simulink subsystem "Controller"  (R2024b)
settings: Solver=VariableStepAuto  StartTime=0.0  StopTime=10.0  RelTol=1e-3
undefined symbols (not defined in the file or in its folder): flight_mode, Parameters, References
libraries: sharedtransform x13, eeGeneralControl x10, simulink x5, aerolibutil x2
(part 3 of 3)

== matlab function Controller/Subsystem/OLD/position_control + autonomous/If Action Subsystem/Attitude + Position FF control/MATLAB Function1 ==
  data: T_des output; p_ref input; att_dir_correction_from_pos_ output; v_ref input; a_ref input; K_pos input; K_pos_int input; K_vel input; K_acc input; pi input; vi input; ai input; q input; p_fb_int input; p_fb_out output
function [T_des, att_dir_correction_from_pos_, p_fb_out] = pos_FF_control(...
    p_ref, v_ref, a_ref, ...
    K_pos, K_pos_int, K_vel, K_acc,...
    pi, vi, ai, q,...
    p_fb_int)

%% inputs %%
p_ref_ = p_ref(1:3,1);      %[m] reference position (in inertial frame)
v_ref_ = v_ref(1:3,1);      %[m/s] reference velocity (in inertial frame)
a_ref_ = a_ref(1:3,1);      %[m/s2] reference acceleration (in inertial frame)
% psi_ref_ = psi_ref(1,1);    %[rad] reference heading

% J_ = J(1:3,1:3);            % moment of inertia matrix
% D_ = diag(D(1,1:3));        % drag coefficient
% g_ = g(1,1);                %[m/s2] acceleration due to gravity
K_pos_ = ...
    K_pos(1:3,1:3);     % position controller gains
K_pos_int_ = ...
    K_pos_int(1:3,1:3); % position controller integral gains
K_vel_ = ...
    K_vel(1:3,1:3);     % velocity controller gains
K_acc_ = ...
    K_acc(1:3,1:3);     % acceleration controller gains
% K_att_ = ...
%     K_att(1:3,1:3);     % attitude controller gains
% K_omega_ = ...
    % K_omega(1:3,1:3);   % body rate controller gains
% A_ = A(1:3,1:3);            % velocity-dependant drag coefficients
% B_ = B(1:3,1:3);            % omega-dependant drag coefficients
% k_h_ = k_h(1,1);            % constant for a quadratic velocity-dependent input disturbance

% q_ref_ = q_ref(1,1:4);      % reference attitude quaternian
% omega_ref_ = ...
%     omega_ref(1:3,1);       %[rad/s] reference body rates
% omega_dot_ref_ = ...
%     omega_dot_ref(1:3,1);   %[rad/s2] reference body rotational acceleration
% Tau_ref_ = Tau_ref(1:3,1);  %[N-m] reference torque
% T_ref_ = T_ref(1,1);        %[N] reference collective thrust

pi_ = pi(1:3,1);            %[m] estimated position (in inertial frame)
vi_ = vi(1:3,1);            %[m/s] estimated velocity (in inertial frame)
ai_ = ai(1:3,1);            %[m/s2] estimated acceleration (in inertial frame)
q_ = q(1,1:4);              %[qw qx qy qz] estimated quaternian attitude
% omega_ = omega(1:3,1);      %[rad/s] estimated body rotation rates
% tau_gyro_ = ...
    % tau_gyro(1:3,1);        %[N-m] estimated gyroscopic torque due to motor spin

p_fb_int_ = p_fb_int(1:3,1); %integral of the position feedback term  

%% outputs %%
% T_des = 0;                  %[N] desired thrust
% Tau_des = zeros(3,1);       %[N-m] desired torque
% p_fb = zeros(3,1);
% v_fb = zeros(3,1);
% a_fb_ = zeros(3,1);

% att_fb = zeros(3,1);
% omega_fb = zeros(3,1);
% omega_dot_des = zeros(3,1);
T_des = 0;
p_fb_out = zeros(3,1); %we will integrate this

%% Positon Control %%
MAX_XYZ_POS_ERR = 10.0;
MAX_XYZ_VEL_ERR = 5.0;
MAX_XYZ_ACC_ERR = 3;


%feedback control:
p_fb_ = (p_ref_ - pi_);
p_fb_out(:) = p_fb_(:);
p_fb_ = K_pos_ * (saturate_err_vec_(p_fb_, -MAX_XYZ_POS_ERR, MAX_XYZ_POS_ERR)) + K_pos_int_*p_fb_int_;

v_fb_ = (v_ref_ - vi_);
v_fb_ = K_vel_ * (saturate_err_vec_(v_fb_, -MAX_XYZ_VEL_ERR, MAX_XYZ_VEL_ERR));

a_fb_ = (a_ref_ - ai_);
a_fb_ = K_acc_ * (saturate_err_vec_(a_fb_, -MAX_XYZ_ACC_ERR, MAX_XYZ_ACC_ERR));

%feedback component:
att_dir_correction_from_pos_ = a_fb_ + v_fb_ + p_fb_; %from position controller

%thrust feedback:
T_des(1) = [att_dir_correction_from_pos_(1),att_dir_correction_from_pos_(2),att_dir_correction_from_pos_(3)]*lib.math.quatrotate(q_, [0;0;-1]);

end

function out = saturate_err_vec_(in, out_min, out_max)
    n = length(in);
    if ~isequal(length(out_min),n)
        out_min_ = out_min(1)*ones(1,n);
    else
        out_min_ = out_min(:)';
    end
    if ~isequal(length(out_max),n)
        out_max_ = out_max(1)*ones(1,n);
    else
        out_max_ = out_max(:)';
    end
    out = zeros(n,1);
    for i = 1:n
        out(i) = saturate_err__(in(i), out_min_(i), out_max_(i));
    end

    function out = saturate_err__(in, out_min, out_max)
        in_ = in(1);
        if in_ > out_max
            out = 1;
            return;
        elseif in_ < out_min
            out = -1;
            return;
        else
            out = in_ / (out_max - out_min);
            return;
        end
    end
end
function out = sqrt_ctr_(in)
    out = sign(in) .*sqrt(abs(in));
end
function out = nthrt_ctr_(in)
    out = sign(in) .*nthroot(abs(in),3);
end

== matlab function Controller/Subsystem/OLD/position_control + autonomous/If Action Subsystem/Attitude + Position FF control/MATLAB Function2 ==
  data: omega_dot_des output; att_dir_correction_from_pos input; q_ref input; omega_ref input; K_att input; K_omega input; q input; omega input
function omega_dot_des  = att_FF_control(...
    att_dir_correction_from_pos, q_ref, omega_ref, ...
    K_att, K_omega,...
    q, omega)%#codegen

%% inputs %%
K_att_ = ...
    K_att(1:3,1:3);     % attitude controller gains
K_omega_ = ...
    K_omega(1:3,1:3);   % body rate controller gains

q_ref_ = q_ref(1,1:4);      % reference attitude quaternian
omega_ref_ = ...
    omega_ref(1:3,1);       %[rad/s] reference body rates
q_ = q(1,1:4);              %[qw qx qy qz] estimated quaternian attitude
omega_ = omega(1:3,1);      %[rad/s] estimated body rotation rates

%% outputs %%
omega_dot_des = zeros(3,1);

%% Attitude Control %%
%extract x and y errors (in inertial frame)
roll_correction_ = [-att_dir_correction_from_pos(1),att_dir_correction_from_pos(2),0]*lib.math.quatrotate(q_, [0;1;0]);
pitch_correction_ =  [-att_dir_correction_from_pos(1),att_dir_correction_from_pos(2),0]*lib.math.quatrotate(q_, [1;0;0]);

% get reference roll pitch and yaw:
[eul_ref_] = lib.math.quat2eul(q_ref_,"ZYX");
roll_ref_ = eul_ref_(3);
pitch_ref_ = eul_ref_(2);
yaw_ref_ = eul_ref_(1);

%get attitude feeback:
eul_rpy_fb_   = manual_att_control(q_, [roll_ref_ + roll_correction_, pitch_ref_ + pitch_correction_, yaw_ref_]);

% add the rate control:
omega_fb_ = sqrt_ctr_(omega_ref_ - omega_);
% omega_fb_ = nthrt_ctr_(omega_ref_ - omega_);
% omega_fb_ = 6*(omega_ref_ - omega_);
omega_dot_des(:) = K_omega_ * omega_fb_(:)  + K_att_ * eul_rpy_fb_(:);
end

function out = sqrt_ctr_(in)
    out = sign(in) .*sqrt(abs(in));
end

== matlab function Controller/Subsystem/OLD/position_control + autonomous/If Action Subsystem/Attitude + Position FF control1/MATLAB Function1 ==
  data: T_des output; p_ref input; omega_dot_des output; v_ref input; a_ref input; psi_ref input; q_ref input; omega_ref input; K_pos input; K_pos_int input; K_vel input; K_acc input; K_att input; K_omega input; pi input; vi input; ai input; q input; omega input; p_fb_int input; p_fb_out output
function [T_des, omega_dot_des, p_fb_out] = att_pos_FF_control(...
    p_ref, v_ref, a_ref, psi_ref, ...
    q_ref, omega_ref, ...
    K_pos, K_pos_int, K_vel, K_acc,...
    K_att, K_omega,...
    pi, vi, ai, q, omega,...
    p_fb_int)

[omega_dot_des, T_des, p_fb_out] = att_pos_FF_control(...
    p_ref, v_ref, a_ref, psi_ref, ...
    q_ref, omega_ref, ...
    K_pos, K_pos_int, K_vel, K_acc,...
    K_att, K_omega,...
    pi, vi, ai, q, omega,...
    p_fb_int);

end

== matlab function Controller/Subsystem/OLD/position_control + autonomous/If Action Subsystem/Attitude + Position FF control2/MATLAB Function1 ==
  data: T_des output; p_ref input; att_dir_correction_from_pos_ output; v_ref input; a_ref input; K_pos input; K_pos_int input; K_vel input; K_acc input; pi input; vi input; ai input; q input; p_fb_int input; p_fb_out output
function [T_des, att_dir_correction_from_pos_, p_fb_out] = pos_FF_control(...
    p_ref, v_ref, a_ref, ...
    K_pos, K_pos_int, K_vel, K_acc,...
    pi, vi, ai, q,...
    p_fb_int)

%% inputs %%
p_ref_ = p_ref(1:3,1);      %[m] reference position (in inertial frame)
v_ref_ = v_ref(1:3,1);      %[m/s] reference velocity (in inertial frame)
a_ref_ = a_ref(1:3,1);      %[m/s2] reference acceleration (in inertial frame)
% psi_ref_ = psi_ref(1,1);    %[rad] reference heading

% J_ = J(1:3,1:3);            % moment of inertia matrix
% D_ = diag(D(1,1:3));        % drag coefficient
% g_ = g(1,1);                %[m/s2] acceleration due to gravity
K_pos_ = ...
    K_pos(1:3,1:3);     % position controller gains
K_pos_int_ = ...
    K_pos_int(1:3,1:3); % position controller integral gains
K_vel_ = ...
    K_vel(1:3,1:3);     % velocity controller gains
K_acc_ = ...
    K_acc(1:3,1:3);     % acceleration controller gains
% K_att_ = ...
%     K_att(1:3,1:3);     % attitude controller gains
% K_omega_ = ...
    % K_omega(1:3,1:3);   % body rate controller gains
% A_ = A(1:3,1:3);            % velocity-dependant drag coefficients
% B_ = B(1:3,1:3);            % omega-dependant drag coefficients
% k_h_ = k_h(1,1);            % constant for a quadratic velocity-dependent input disturbance

% q_ref_ = q_ref(1,1:4);      % reference attitude quaternian
% omega_ref_ = ...
%     omega_ref(1:3,1);       %[rad/s] reference body rates
% omega_dot_ref_ = ...
%     omega_dot_ref(1:3,1);   %[rad/s2] reference body rotational acceleration
% Tau_ref_ = Tau_ref(1:3,1);  %[N-m] reference torque
% T_ref_ = T_ref(1,1);        %[N] reference collective thrust

pi_ = pi(1:3,1);            %[m] estimated position (in inertial frame)
vi_ = vi(1:3,1);            %[m/s] estimated velocity (in inertial frame)
ai_ = ai(1:3,1);            %[m/s2] estimated acceleration (in inertial frame)
q_ = q(1,1:4);              %[qw qx qy qz] estimated quaternian attitude
% omega_ = omega(1:3,1);      %[rad/s] estimated body rotation rates
% tau_gyro_ = ...
    % tau_gyro(1:3,1);        %[N-m] estimated gyroscopic torque due to motor spin

p_fb_int_ = p_fb_int(1:3,1); %integral of the position feedback term  

%% outputs %%
% T_des = 0;                  %[N] desired thrust
% Tau_des = zeros(3,1);       %[N-m] desired torque
% p_fb = zeros(3,1);
% v_fb = zeros(3,1);
% a_fb_ = zeros(3,1);

% att_fb = zeros(3,1);
% omega_fb = zeros(3,1);
% omega_dot_des = zeros(3,1);
T_des = 0;
p_fb_out = zeros(3,1); %we will integrate this

%% Positon Control %%
MAX_XYZ_POS_ERR = 10.0;
MAX_XYZ_VEL_ERR = 5.0;
MAX_XYZ_ACC_ERR = 3;


%feedback control:
p_fb_ = (p_ref_ - pi_);
p_fb_out(:) = p_fb_(:);
p_fb_ = K_pos_ * (saturate_err_vec_(p_fb_, -MAX_XYZ_POS_ERR, MAX_XYZ_POS_ERR)) + K_pos_int_*p_fb_int_;

v_fb_ = (v_ref_ - vi_);
v_fb_ = K_vel_ * (saturate_err_vec_(v_fb_, -MAX_XYZ_VEL_ERR, MAX_XYZ_VEL_ERR));

a_fb_ = (a_ref_ - ai_);
a_fb_ = K_acc_ * (saturate_err_vec_(a_fb_, -MAX_XYZ_ACC_ERR, MAX_XYZ_ACC_ERR));

%feedback component:
att_dir_correction_from_pos_ = a_fb_ + v_fb_ + p_fb_; %from position controller

%thrust feedback:
T_des(1) = [att_dir_correction_from_pos_(1),att_dir_correction_from_pos_(2),att_dir_correction_from_pos_(3)]*lib.math.quatrotate(q_, [0;0;-1]);

end

function out = saturate_err_vec_(in, out_min, out_max)
    n = length(in);
    if ~isequal(length(out_min),n)
        out_min_ = out_min(1)*ones(1,n);
    else
        out_min_ = out_min(:)';
    end
    if ~isequal(length(out_max),n)
        out_max_ = out_max(1)*ones(1,n);
    else
        out_max_ = out_max(:)';
    end
    out = zeros(n,1);
    for i = 1:n
        out(i) = saturate_err__(in(i), out_min_(i), out_max_(i));
    end

    function out = saturate_err__(in, out_min, out_max)
        in_ = in(1);
        if in_ > out_max
            out = 1;
            return;
        elseif in_ < out_min
            out = -1;
            return;
        else
            out = in_ / (out_max - out_min);
            return;
        end
    end
end
function out = sqrt_ctr_(in)
    out = sign(in) .*sqrt(abs(in));
end
function out = nthrt_ctr_(in)
    out = sign(in) .*nthroot(abs(in),3);
end

== matlab function Controller/Subsystem/OLD/position_control + autonomous/If Action Subsystem/Attitude + Position FF control2/MATLAB Function2 ==
  data: omega_dot_des output; att_dir_correction_from_pos input; q_ref input; omega_ref input; K_att input; K_omega input; q input; omega input
function omega_dot_des  = att_FF_control(...
    att_dir_correction_from_pos, q_ref, omega_ref, ...
    K_att, K_omega,...
    q, omega)%#codegen

%% inputs %%
K_att_ = ...
    K_att(1:3,1:3);     % attitude controller gains
K_omega_ = ...
    K_omega(1:3,1:3);   % body rate controller gains

q_ref_ = q_ref(1,1:4);      % reference attitude quaternian
omega_ref_ = ...
    omega_ref(1:3,1);       %[rad/s] reference body rates
q_ = q(1,1:4);              %[qw qx qy qz] estimated quaternian attitude
omega_ = omega(1:3,1);      %[rad/s] estimated body rotation rates

%% outputs %%
omega_dot_des = zeros(3,1);

%% Attitude Control %%
%extract x and y errors (in inertial frame)
roll_correction_ = [-att_dir_correction_from_pos(1),att_dir_correction_from_pos(2),0]*lib.math.quatrotate(q_, [0;1;0]);
pitch_correction_ =  [-att_dir_correction_from_pos(1),att_dir_correction_from_pos(2),0]*lib.math.quatrotate(q_, [1;0;0]);

% get reference roll pitch and yaw:
[eul_ref_] = lib.math.quat2eul(q_ref_,"ZYX");
roll_ref_ = eul_ref_(3);
pitch_ref_ = eul_ref_(2);
yaw_ref_ = eul_ref_(1);

%get attitude feeback:
% eul_rpy_fb_   = manual_att_control(q_, [roll_ref_ + roll_correction_, pitch_ref_ + pitch_correction_, yaw_ref_]);

q_ref_ = eul2quat([roll_ref_ + roll_correction_, pitch_ref_ + pitch_correction_, yaw_ref_], "ZYX");
rate_ref = att_quat_control(q_, q_ref_, omega_ref_(3), diag(K_att_), [1000, 1000, 1000]);

% add the rate control:
omega_fb_ = (omega_ref_ + rate_ref - omega_);
% omega_fb_ = nthrt_ctr_(omega_ref_ - omega_);
% omega_fb_ = 6*(omega_ref_ - omega_);
omega_dot_des(:) = K_omega_ * omega_fb_(:);
end

function out = sqrt_ctr_(in)
    out = sign(in) .*sqrt(abs(in));
end

== matlab function Controller/Subsystem/OLD/position_control + autonomous/K-matrix control/K-matrix-control/MATLAB Function2 ==
  data: pi input; Tau_des output; vi input; q input; omega input; T_des output; K input; R_ref input; V_ref input; att_ref input; w_ref input; T_ref input; Tau_ref input; p_fb_int input; p_fb_out output
function [Tau_des, T_des, p_fb_out] = LQR_control(...
    pi, vi, q, omega, K,...
    R_ref, V_ref, att_ref, w_ref,...
    T_ref, Tau_ref, p_fb_int)
[Tau_des, T_des, p_fb_out] = LQR_control(...
    pi, vi, q, omega, K,...
    R_ref, V_ref, att_ref, w_ref,...
    T_ref, Tau_ref, p_fb_int);
end

== matlab function Controller/Subsystem/New/Translational Motion Feedback Selector/Switch Case Action Subsystem/Translational Motion Control/MATLAB Function1 ==
  data: thrust_ref output; pos_ref input; vel_ref input; acc_ref input; K_pos input; K_pos_int input; K_vel input; K_acc input; pos_i input; vel_i input; acc_i input; GC input; ff_thrust input; m input; g input; MAX_VEL_HORIZONTAL input; MAX_VEL_VERTICAL input; MAX_TILT_RAD input; MIN_TH input; MAX_TH input; dt input; vel_int input; vel_int_out output
function [thrust_ref, vel_int_out] = pos_FF_control(...
    pos_ref, vel_ref, acc_ref, ...
    K_pos, K_pos_int, K_vel, K_acc,...
    pos_i, vel_i, acc_i, ...
    GC, ff_thrust, m, g, MAX_VEL_HORIZONTAL, MAX_VEL_VERTICAL, MAX_TILT_RAD, MIN_TH, MAX_TH,...
    dt, vel_int)

%% inputs %%
pos_ref_ = pos_ref(1:3,1);      %[m] reference position (in inertial frame)
vel_ref_ = vel_ref(1:3,1);      %[m/s] reference velocity (in inertial frame)
acc_ref_ = acc_ref(1:3,1);      %[m/s2] reference acceleration (in inertial frame)

K_pos_ = ...
    K_pos(1:3,1:3);     % position controller gains
K_vel_int_ = ...
    K_pos_int(1:3,1:3); % velocity controller integral gains
K_vel_ = ...
    K_vel(1:3,1:3);     % velocity controller gains
K_acc_ = ...
    K_acc(1:3,1:3);     % acceleration controller gains

pos_i_ = pos_i(1:3,1);            %[m] estimated position (in inertial frame)
vel_i_ = vel_i(1:3,1);            %[m/s] estimated velocity (in inertial frame)
acc_i_ = acc_i(1:3,1);            %[m/s2] estimated acceleration (in inertial frame)
% q_ = q(1,1:4);              %[qw qx qy qz] estimated quaternian attitude

vel_int_ = vel_int(1:3,1); %integral of the position feedback term  

GC_ = GC(1);

%% outputs %%
% T_des = 0;                  %[N] desired thrust
vel_int_out = zeros(3,1); %we will integrate this
thrust_ref = zeros(3,1);

% MAX_VEL_HORIZONTAL = 5.0;
% MAX_VEL_VERTICAL = 5.0;
% MAX_TILT_RAD = 30*pi/180;
% MIN_TH = 0.05*4*MAX_THRUST;
% MAX_TH = 0.9*4*MAX_THRUST;


%% Position Feedback Control %%
p_fb_ = K_pos_ * (pos_ref_ - pos_i_);
vel_ref_ = lib.math.addifnotnan(vel_ref_, p_fb_);
p_fb_ = lib.math.setzeroifnan(p_fb_);
vel_ref_([1,2]) = lib.math.constrain2D(p_fb_, vel_ref_ - p_fb_, MAX_VEL_HORIZONTAL);
vel_ref_(3) = lib.math.constrain(vel_ref_(3), -MAX_VEL_VERTICAL, MAX_VEL_VERTICAL);

%% Velocity Feedback Control %%
v_error_ = (vel_ref_ - vel_i_);
if GC_ %disable interator term if in ground contact (should already be zero, but just in case)
    acc_sp_velocity = K_vel_*v_error_ + K_acc_ * (acc_ref_ - acc_i_);
else
    acc_sp_velocity = K_vel_*v_error_ + K_vel_int_*vel_int_ + K_acc_ * (acc_ref_ - acc_i_);
end
acc_ref_ = lib.math.setzeroifnan(acc_sp_velocity);
% acc_ref_ = lib.math.addifnotnan(acc_ref_, acc_sp_velocity);

% Acceleration / thrust (vertical):
%Assume standard acceleration due to gravity in vertical direction for attitude generation
body_z = [-acc_ref_(1); acc_ref_(2); g];
body_z = body_z / norm(body_z);
body_z = lib.math.limitTilt(body_z, [0;0;1], MAX_TILT_RAD);

%Scale thrust assuming hover thrust produces standard gravity
% hover_thrust = -m*g;
collective_thrust = acc_ref_(3) * m  - ff_thrust; %%ff thrust is scalar and always positive
%Project thrust to planned body attitude
collective_thrust = collective_thrust/dot([0;0;1], body_z);
collective_thrust = min(collective_thrust, -MIN_TH);
thr_sp = body_z * collective_thrust;

% Integrator anti-windup in vertical direction
if ((thr_sp(3) >= -MIN_TH && v_error_(3) >= 0.0) || ...
    (thr_sp(3) <= -MAX_TH && v_error_(3) <= 0.0)) 
	v_error_(3) = 0.0;
end

% Saturate maximal vertical thrust
thr_sp(3) = max(thr_sp(3), -MAX_TH);

% Get allowed horizontal thrust after prioritizing vertical control
thrust_max_squared = MAX_TH * MAX_TH;
thrust_z_squared = thr_sp(3) * thr_sp(3);
thrust_max_xy_squared = thrust_max_squared - thrust_z_squared;
thrust_max_xy = 0;

if (thrust_max_xy_squared > 0)
	thrust_max_xy = sqrt(thrust_max_xy_squared);
end

% Saturate thrust in horizontal direction
thrust_sp_xy = [thr_sp(1); thr_sp(2)];
thrust_sp_xy_norm = norm(thrust_sp_xy);

if (thrust_sp_xy_norm > thrust_max_xy)
	thr_sp([1,2]) = thrust_sp_xy / thrust_sp_xy_norm * thrust_max_xy;
end

if GC_ %disable interator term if in ground contact
    vel_int_out(:) = zeros(3,1);
else
    % Use tracking Anti-Windup for horizontal direction: during saturation, the integrator is used to unsaturate the output
    % see Anti-Reset Windup for PID controllers, L.Rundqwist, 1990
    % acc_sp_xy_limited = thr_sp([1,2]) / m;
    % arw_gain = [2.0 / K_vel_(1,1); 2.0 / K_vel_(2,2)];
    v_error_([1,2]) = v_error_([1,2]);% - (arw_gain .* (acc_ref_([1,2]) - acc_sp_xy_limited));
    
    % Make sure integral doesn't get NAN
    v_error_ = lib.math.setzeroifnan(v_error_);
    % Update integral part of velocity control
    vel_int_ = vel_int_ + K_vel_int_*v_error_ * dt;
    
    
    % limit thrust integral
    vel_int_(3) = min(abs(vel_int_(3)), g) * sign(vel_int_(3));
    
    vel_int_out(:) = vel_int_(:);
end

thrust_ref(:) = thr_sp(:); %from position controller
end

== matlab function Controller/Subsystem/New/Translational Motion Feedback Selector/Switch Case Action Subsystem1/Translational Motion Control/MATLAB Function ==
  data: body_z input; q_sp output; yaw_sp input
function q_sp = fcn(body_z, yaw_sp)
body_z([1,3]) = -body_z([1,3]);
q_sp = lib.math.bodyzToAttitude(body_z, yaw_sp);
end

== matlab function Controller/Subsystem/OLD/manual control (attitude only)/Subsystem/Subsystem2/MATLAB Function2 ==
  data: q input; att_ref input; rpy_rate_fb output
function rpy_rate_fb   = manual_att_control(q, att_ref)
rpy_rate_fb   = manual_att_control(q, att_ref);
end
